simulink library "PD_Controller_Lib"  (R2018b)
settings: Solver=VariableStepAuto  StartTime=0.0  StopTime=10.0  RelTol=1e-3
undefined symbols (not defined in the file or in its folder): fswParams
settings Model: Creator=devantormey  LastModifiedBy=Taylor

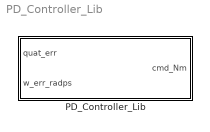
== system PD_Controller_Lib ==
  PD_Controller_Lib : Subsystem  TreatAsAtomicUnit=on
      settings: RTWFcnNameOpts=Use subsystem name  RTWFileNameOpts=Use subsystem name

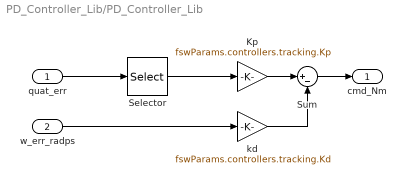
== system PD_Controller_Lib/PD_Controller_Lib ==
  quat_err : Inport
  w_err_radps : Inport  Port=2
  Kp : Gain  Gain=fswParams.controllers.tracking.Kp
  Selector : Selector  InputPortWidth=4  IndexOptions=Index vector (dialog)  Indices=[2 3 4]  OutputSizes=1
  Sum : Sum  Inputs=|+-
  kd : Gain  Gain=fswParams.controllers.tracking.Kd
  cmd_Nm : Outport
  wires:
  Kp/1 -> Sum/1
  kd/1 -> Sum/2
  Sum/1 -> cmd_Nm/1
  quat_err/1 -> Selector/1
  w_err_radps/1 -> kd/1
  Selector/1 -> Kp/1
